simulink model "GalacticSoupPhysical"  (R2025b)
settings: Solver=VariableStepAuto  StartTime=0.0  StopTime=10.0  RelTol=1e-3
settings Model: DataDictionary=GalacticSoupPhysicalInterfaces.sldd  Creator=sarah  LastModifiedBy=sarah

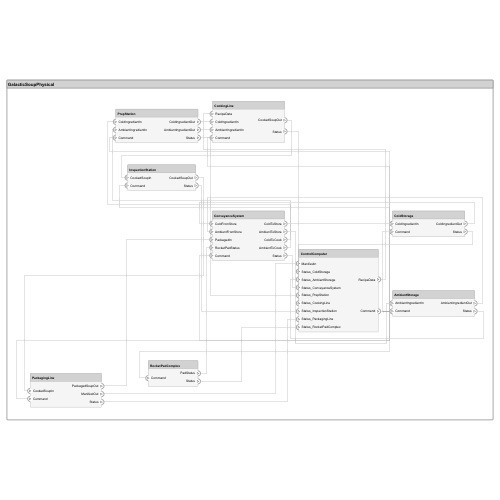
[thumbnail: Simulink's stored preview of the top-level diagram]
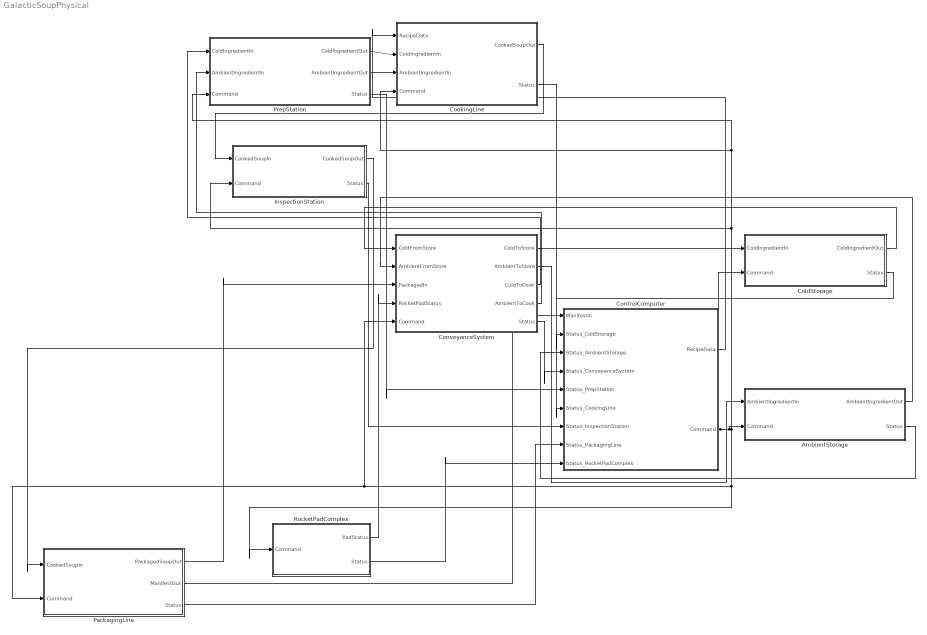
== system GalacticSoupPhysical ==
  AmbientStorage : Subsystem
      settings: PortSchema="{\"entries\":[{\"content\":{\"headerSize\":26,\"margin\":15,\"minimumSpacing\":25,\"sides\":[{\"content\":{\"connectorIds\":[\"In1\",\"In2\"]},\"type\":\"ConnectorPlacement.EquallySpacedRectSide\",\"uuid\":\"47548036-a6c3-440f-b573-2a4e753e82ae\"},{\"content\":{\"connectorIds\":[\"Out1\",\"Out2\"],\"side\":\"RIGHT\"},\"type\":\"ConnectorPlacement.EquallySpacedRectSide\",\"uuid\":\"ab096620-2054-4429-8520-52cfe6541bb8\"},{\"content\":{\"side\":\"TOP\"},\"type\":\"ConnectorPlacement.EquallySpacedRectSide\",\"uuid\":\"6e18e29c-ba68-48ca-8847-f496b38e15b5\"}]},\"type\":\"ConnectorPlacement.EquallySpacedConnector\",\"uuid\":\"7233fc04-a641-40d9-8870-909b934a9733\"}],\"packageUris\":[\"http://schema.mathworks.com/mf0/Connector/R2020b\"],\"version\":\"1.0\"}"
  ColdStorage : Subsystem
      settings: PortSchema="{\"entries\":[{\"content\":{\"headerSize\":26,\"margin\":15,\"minimumSpacing\":25,\"sides\":[{\"content\":{\"connectorIds\":[\"In1\",\"In2\"]},\"type\":\"ConnectorPlacement.EquallySpacedRectSide\",\"uuid\":\"47548036-a6c3-440f-b573-2a4e753e82ae\"},{\"content\":{\"connectorIds\":[\"Out1\",\"Out2\"],\"side\":\"RIGHT\"},\"type\":\"ConnectorPlacement.EquallySpacedRectSide\",\"uuid\":\"ab096620-2054-4429-8520-52cfe6541bb8\"},{\"content\":{\"side\":\"TOP\"},\"type\":\"ConnectorPlacement.EquallySpacedRectSide\",\"uuid\":\"6e18e29c-ba68-48ca-8847-f496b38e15b5\"}]},\"type\":\"ConnectorPlacement.EquallySpacedConnector\",\"uuid\":\"7233fc04-a641-40d9-8870-909b934a9733\"}],\"packageUris\":[\"http://schema.mathworks.com/mf0/Connector/R2020b\"],\"version\":\"1.0\"}"
  ControlComputer : Subsystem
      settings: PortSchema="{\"entries\":[{\"content\":{\"headerSize\":26,\"margin\":15,\"minimumSpacing\":25,\"sides\":[{\"content\":{\"connectorIds\":[\"In1\",\"In2\",\"In3\",\"In4\",\"In5\",\"In6\",\"In7\",\"In8\",\"In9\"]},\"type\":\"ConnectorPlacement.EquallySpacedRectSide\",\"uuid\":\"47548036-a6c3-440f-b573-2a4e753e82ae\"},{\"content\":{\"connectorIds\":[\"Out1\",\"Out2\"],\"side\":\"RIGHT\"},\"type\":\"ConnectorPlacement.EquallySpacedRectSide\",\"uuid\":\"ab096620-2054-4429-8520-52cfe6541bb8\"},{\"content\":{\"side\":\"TOP\"},\"type\":\"ConnectorPlacement.EquallySpacedRectSide\",\"uuid\":\"6e18e29c-ba68-48ca-8847-f496b38e15b5\"}]},\"type\":\"ConnectorPlacement.EquallySpacedConnector\",\"uuid\":\"7233fc04-a641-40d9-8870-909b934a9733\"}],\"packageUris\":[\"http://schema.mathworks.com/mf0/Connector/R2020b\"],\"version\":\"1.0\"}"
  ConveyanceSystem : Subsystem
      settings: PortSchema="{\"entries\":[{\"content\":{\"headerSize\":26,\"margin\":15,\"minimumSpacing\":25,\"sides\":[{\"content\":{\"connectorIds\":[\"In1\",\"In2\",\"In3\",\"In4\",\"In5\"]},\"type\":\"ConnectorPlacement.EquallySpacedRectSide\",\"uuid\":\"47548036-a6c3-440f-b573-2a4e753e82ae\"},{\"content\":{\"connectorIds\":[\"Out1\",\"Out2\",\"Out3\",\"Out4\",\"Out5\"],\"side\":\"RIGHT\"},\"type\":\"ConnectorPlacement.EquallySpacedRectSide\",\"uuid\":\"ab096620-2054-4429-8520-52cfe6541bb8\"},{\"content\":{\"side\":\"TOP\"},\"type\":\"ConnectorPlacement.EquallySpacedRectSide\",\"uuid\":\"6e18e29c-ba68-48ca-8847-f496b38e15b5\"}]},\"type\":\"ConnectorPlacement.EquallySpacedConnector\",\"uuid\":\"7233fc04-a641-40d9-8870-909b934a9733\"}],\"packageUris\":[\"http://schema.mathworks.com/mf0/Connector/R2020b\"],\"version\":\"1.0\"}"
  CookingLine : Subsystem
      settings: PortSchema="{\"entries\":[{\"content\":{\"headerSize\":26,\"margin\":15,\"minimumSpacing\":25,\"sides\":[{\"content\":{\"connectorIds\":[\"In1\",\"In2\",\"In3\",\"In4\"]},\"type\":\"ConnectorPlacement.EquallySpacedRectSide\",\"uuid\":\"47548036-a6c3-440f-b573-2a4e753e82ae\"},{\"content\":{\"connectorIds\":[\"Out1\",\"Out2\"],\"side\":\"RIGHT\"},\"type\":\"ConnectorPlacement.EquallySpacedRectSide\",\"uuid\":\"ab096620-2054-4429-8520-52cfe6541bb8\"},{\"content\":{\"side\":\"TOP\"},\"type\":\"ConnectorPlacement.EquallySpacedRectSide\",\"uuid\":\"6e18e29c-ba68-48ca-8847-f496b38e15b5\"}]},\"type\":\"ConnectorPlacement.EquallySpacedConnector\",\"uuid\":\"7233fc04-a641-40d9-8870-909b934a9733\"}],\"packageUris\":[\"http://schema.mathworks.com/mf0/Connector/R2020b\"],\"version\":\"1.0\"}"
  InspectionStation : Subsystem
      settings: PortSchema="{\"entries\":[{\"content\":{\"headerSize\":26,\"margin\":15,\"minimumSpacing\":25,\"sides\":[{\"content\":{\"connectorIds\":[\"In1\",\"In2\"]},\"type\":\"ConnectorPlacement.EquallySpacedRectSide\",\"uuid\":\"47548036-a6c3-440f-b573-2a4e753e82ae\"},{\"content\":{\"connectorIds\":[\"Out1\",\"Out2\"],\"side\":\"RIGHT\"},\"type\":\"ConnectorPlacement.EquallySpacedRectSide\",\"uuid\":\"ab096620-2054-4429-8520-52cfe6541bb8\"},{\"content\":{\"side\":\"TOP\"},\"type\":\"ConnectorPlacement.EquallySpacedRectSide\",\"uuid\":\"6e18e29c-ba68-48ca-8847-f496b38e15b5\"}]},\"type\":\"ConnectorPlacement.EquallySpacedConnector\",\"uuid\":\"7233fc04-a641-40d9-8870-909b934a9733\"}],\"packageUris\":[\"http://schema.mathworks.com/mf0/Connector/R2020b\"],\"version\":\"1.0\"}"
  PackagingLine : Subsystem
      settings: PortSchema="{\"entries\":[{\"content\":{\"headerSize\":26,\"margin\":15,\"minimumSpacing\":25,\"sides\":[{\"content\":{\"connectorIds\":[\"In1\",\"In2\"]},\"type\":\"ConnectorPlacement.EquallySpacedRectSide\",\"uuid\":\"47548036-a6c3-440f-b573-2a4e753e82ae\"},{\"content\":{\"connectorIds\":[\"Out1\",\"Out2\",\"Out3\"],\"side\":\"RIGHT\"},\"type\":\"ConnectorPlacement.EquallySpacedRectSide\",\"uuid\":\"ab096620-2054-4429-8520-52cfe6541bb8\"},{\"content\":{\"side\":\"TOP\"},\"type\":\"ConnectorPlacement.EquallySpacedRectSide\",\"uuid\":\"6e18e29c-ba68-48ca-8847-f496b38e15b5\"}]},\"type\":\"ConnectorPlacement.EquallySpacedConnector\",\"uuid\":\"7233fc04-a641-40d9-8870-909b934a9733\"}],\"packageUris\":[\"http://schema.mathworks.com/mf0/Connector/R2020b\"],\"version\":\"1.0\"}"
  PrepStation : Subsystem
      settings: PortSchema="{\"entries\":[{\"content\":{\"headerSize\":26,\"margin\":15,\"minimumSpacing\":25,\"sides\":[{\"content\":{\"connectorIds\":[\"In1\",\"In2\",\"In3\"]},\"type\":\"ConnectorPlacement.EquallySpacedRectSide\",\"uuid\":\"47548036-a6c3-440f-b573-2a4e753e82ae\"},{\"content\":{\"connectorIds\":[\"Out1\",\"Out2\",\"Out3\"],\"side\":\"RIGHT\"},\"type\":\"ConnectorPlacement.EquallySpacedRectSide\",\"uuid\":\"ab096620-2054-4429-8520-52cfe6541bb8\"},{\"content\":{\"side\":\"TOP\"},\"type\":\"ConnectorPlacement.EquallySpacedRectSide\",\"uuid\":\"6e18e29c-ba68-48ca-8847-f496b38e15b5\"}]},\"type\":\"ConnectorPlacement.EquallySpacedConnector\",\"uuid\":\"7233fc04-a641-40d9-8870-909b934a9733\"}],\"packageUris\":[\"http://schema.mathworks.com/mf0/Connector/R2020b\"],\"version\":\"1.0\"}"
  RocketPadComplex : Subsystem
      settings: PortSchema="{\"entries\":[{\"content\":{\"headerSize\":26,\"margin\":15,\"minimumSpacing\":25,\"sides\":[{\"content\":{\"connectorIds\":[\"In1\"]},\"type\":\"ConnectorPlacement.EquallySpacedRectSide\",\"uuid\":\"47548036-a6c3-440f-b573-2a4e753e82ae\"},{\"content\":{\"connectorIds\":[\"Out1\",\"Out2\"],\"side\":\"RIGHT\"},\"type\":\"ConnectorPlacement.EquallySpacedRectSide\",\"uuid\":\"ab096620-2054-4429-8520-52cfe6541bb8\"},{\"content\":{\"side\":\"TOP\"},\"type\":\"ConnectorPlacement.EquallySpacedRectSide\",\"uuid\":\"6e18e29c-ba68-48ca-8847-f496b38e15b5\"}]},\"type\":\"ConnectorPlacement.EquallySpacedConnector\",\"uuid\":\"7233fc04-a641-40d9-8870-909b934a9733\"}],\"packageUris\":[\"http://schema.mathworks.com/mf0/Connector/R2020b\"],\"version\":\"1.0\"}"
  wires:
  RocketPadComplex/2(Status) -> ControlComputer/9(Status_RocketPadComplex)
  PrepStation/2(AmbientIngredientOut) -> CookingLine/3(AmbientIngredientIn)
  InspectionStation/1(CookedSoupOut) -> PackagingLine/1(CookedSoupIn)
  InspectionStation/2(Status) -> ControlComputer/7(Status_InspectionStation)
  PackagingLine/3(Status) -> ControlComputer/8(Status_PackagingLine)
  PackagingLine/1(PackagedSoupOut) -> ConveyanceSystem/3(PackagedIn)
  PackagingLine/2(ManifestOut) -> ControlComputer/1(ManifestIn)
  PrepStation/1(ColdIngredientOut) -> CookingLine/2(ColdIngredientIn)
  PrepStation/3(Status) -> ControlComputer/5(Status_PrepStation)
  RocketPadComplex/1(PadStatus) -> ConveyanceSystem/4(RocketPadStatus)
  CookingLine/1(CookedSoupOut) -> InspectionStation/1(CookedSoupIn)
  CookingLine/2(Status) -> ControlComputer/6(Status_CookingLine)
  ConveyanceSystem/1(ColdToStore) -> ColdStorage/1(ColdIngredientIn)
  ConveyanceSystem/2(AmbientToStore) -> AmbientStorage/1(AmbientIngredientIn)
  ConveyanceSystem/4(AmbientToCook) -> PrepStation/2(AmbientIngredientIn)
  ConveyanceSystem/3(ColdToCook) -> PrepStation/1(ColdIngredientIn)
  ConveyanceSystem/5(Status) -> ControlComputer/4(Status_ConveyanceSystem)
  ControlComputer/2(Command) -> PackagingLine/2(Command), ConveyanceSystem/5(Command), RocketPadComplex/1(Command), CookingLine/4(Command), PrepStation/3(Command), InspectionStation/2(Command), AmbientStorage/2(Command), ColdStorage/2(Command)
  ControlComputer/1(RecipeData) -> CookingLine/1(RecipeData)
  ColdStorage/1(ColdIngredientOut) -> ConveyanceSystem/1(ColdFromStore)
  ColdStorage/2(Status) -> ControlComputer/2(Status_ColdStorage)
  AmbientStorage/1(AmbientIngredientOut) -> ConveyanceSystem/2(AmbientFromStore)
  AmbientStorage/2(Status) -> ControlComputer/3(Status_AmbientStorage)

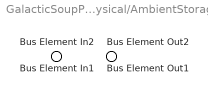
== system GalacticSoupPhysical/AmbientStorage ==
  Bus Element In1 : Inport  PortName=AmbientIngredientIn
  Bus Element In2 : Inport  Port=2  PortName=Command
  Bus Element Out1 : Outport  PortName=AmbientIngredientOut
  Bus Element Out2 : Outport  Port=2  PortName=Status

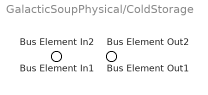
== system GalacticSoupPhysical/ColdStorage ==
  Bus Element In1 : Inport  PortName=ColdIngredientIn
  Bus Element In2 : Inport  Port=2  PortName=Command
  Bus Element Out1 : Outport  PortName=ColdIngredientOut
  Bus Element Out2 : Outport  Port=2  PortName=Status

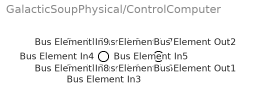
== system GalacticSoupPhysical/ControlComputer ==
  Bus Element In1 : Inport  PortName=ManifestIn
  Bus Element In2 : Inport  Port=2  PortName=Status_ColdStorage
  Bus Element In3 : Inport  Port=3  PortName=Status_AmbientStorage
  Bus Element In4 : Inport  Port=4  PortName=Status_ConveyanceSystem
  Bus Element In5 : Inport  Port=5  PortName=Status_PrepStation
  Bus Element In6 : Inport  Port=6  PortName=Status_CookingLine
  Bus Element In7 : Inport  Port=7  PortName=Status_InspectionStation
  Bus Element In8 : Inport  Port=8  PortName=Status_PackagingLine
  Bus Element In9 : Inport  Port=9  PortName=Status_RocketPadComplex
  Bus Element Out1 : Outport  PortName=RecipeData
  Bus Element Out2 : Outport  Port=2  PortName=Command

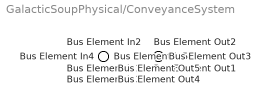
== system GalacticSoupPhysical/ConveyanceSystem ==
  Bus Element In1 : Inport  PortName=ColdFromStore
  Bus Element In2 : Inport  Port=2  PortName=AmbientFromStore
  Bus Element In3 : Inport  Port=3  PortName=PackagedIn
  Bus Element In4 : Inport  Port=4  PortName=RocketPadStatus
  Bus Element In5 : Inport  Port=5  PortName=Command
  Bus Element Out1 : Outport  PortName=ColdToStore
  Bus Element Out2 : Outport  Port=2  PortName=AmbientToStore
  Bus Element Out3 : Outport  Port=3  PortName=ColdToCook
  Bus Element Out4 : Outport  Port=4  PortName=AmbientToCook
  Bus Element Out5 : Outport  Port=5  PortName=Status

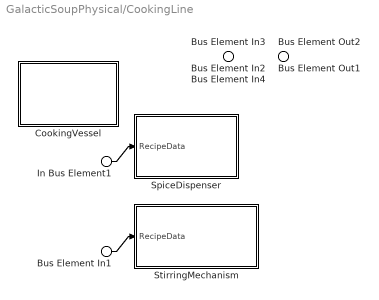
== system GalacticSoupPhysical/CookingLine ==
  Bus Element In1 : Inport  PortName=RecipeData
  In Bus Element1 : Inport  PortName=RecipeData
  Bus Element In2 : Inport  Port=2  PortName=ColdIngredientIn
  Bus Element In3 : Inport  Port=3  PortName=AmbientIngredientIn
  Bus Element In4 : Inport  Port=4  PortName=Command
  CookingVessel : Subsystem
      settings: PortSchema="{\"entries\":[{\"content\":{\"headerSize\":26,\"margin\":15,\"minimumSpacing\":25,\"sides\":[{\"content\":{},\"type\":\"ConnectorPlacement.EquallySpacedRectSide\",\"uuid\":\"47548036-a6c3-440f-b573-2a4e753e82ae\"},{\"content\":{\"side\":\"RIGHT\"},\"type\":\"ConnectorPlacement.EquallySpacedRectSide\",\"uuid\":\"ab096620-2054-4429-8520-52cfe6541bb8\"},{\"content\":{\"side\":\"TOP\"},\"type\":\"ConnectorPlacement.EquallySpacedRectSide\",\"uuid\":\"6e18e29c-ba68-48ca-8847-f496b38e15b5\"}]},\"type\":\"ConnectorPlacement.EquallySpacedConnector\",\"uuid\":\"7233fc04-a641-40d9-8870-909b934a9733\"}],\"packageUris\":[\"http://schema.mathworks.com/mf0/Connector/R2020b\"],\"version\":\"1.0\"}"
  SpiceDispenser : Subsystem
      settings: PortSchema="{\"entries\":[{\"content\":{\"headerSize\":26,\"margin\":15,\"minimumSpacing\":25,\"sides\":[{\"content\":{\"connectorIds\":[\"In1\"]},\"type\":\"ConnectorPlacement.EquallySpacedRectSide\",\"uuid\":\"47548036-a6c3-440f-b573-2a4e753e82ae\"},{\"content\":{\"side\":\"RIGHT\"},\"type\":\"ConnectorPlacement.EquallySpacedRectSide\",\"uuid\":\"ab096620-2054-4429-8520-52cfe6541bb8\"},{\"content\":{\"side\":\"TOP\"},\"type\":\"ConnectorPlacement.EquallySpacedRectSide\",\"uuid\":\"6e18e29c-ba68-48ca-8847-f496b38e15b5\"}]},\"type\":\"ConnectorPlacement.EquallySpacedConnector\",\"uuid\":\"7233fc04-a641-40d9-8870-909b934a9733\"}],\"packageUris\":[\"http://schema.mathworks.com/mf0/Connector/R2020b\"],\"version\":\"1.0\"}"
  StirringMechanism : Subsystem
      settings: PortSchema="{\"entries\":[{\"content\":{\"headerSize\":26,\"margin\":15,\"minimumSpacing\":25,\"sides\":[{\"content\":{\"connectorIds\":[\"In1\"]},\"type\":\"ConnectorPlacement.EquallySpacedRectSide\",\"uuid\":\"47548036-a6c3-440f-b573-2a4e753e82ae\"},{\"content\":{\"side\":\"RIGHT\"},\"type\":\"ConnectorPlacement.EquallySpacedRectSide\",\"uuid\":\"ab096620-2054-4429-8520-52cfe6541bb8\"},{\"content\":{\"side\":\"TOP\"},\"type\":\"ConnectorPlacement.EquallySpacedRectSide\",\"uuid\":\"6e18e29c-ba68-48ca-8847-f496b38e15b5\"}]},\"type\":\"ConnectorPlacement.EquallySpacedConnector\",\"uuid\":\"7233fc04-a641-40d9-8870-909b934a9733\"}],\"packageUris\":[\"http://schema.mathworks.com/mf0/Connector/R2020b\"],\"version\":\"1.0\"}"
  Bus Element Out1 : Outport  PortName=CookedSoupOut
  Bus Element Out2 : Outport  Port=2  PortName=Status
  wires:
  In Bus Element1/1 -> SpiceDispenser/1(RecipeData)
  Bus Element In1/1 -> StirringMechanism/1(RecipeData)

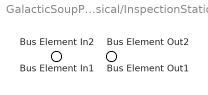
== system GalacticSoupPhysical/InspectionStation ==
  Bus Element In1 : Inport  PortName=CookedSoupIn
  Bus Element In2 : Inport  Port=2  PortName=Command
  Bus Element Out1 : Outport  PortName=CookedSoupOut
  Bus Element Out2 : Outport  Port=2  PortName=Status

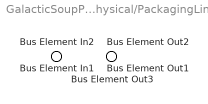
== system GalacticSoupPhysical/PackagingLine ==
  Bus Element In1 : Inport  PortName=CookedSoupIn
  Bus Element In2 : Inport  Port=2  PortName=Command
  Bus Element Out1 : Outport  PortName=PackagedSoupOut
  Bus Element Out2 : Outport  Port=2  PortName=ManifestOut
  Bus Element Out3 : Outport  Port=3  PortName=Status

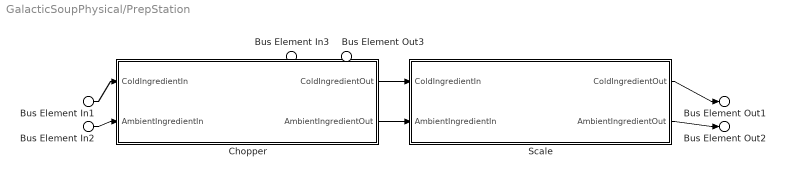
== system GalacticSoupPhysical/PrepStation ==
  Bus Element In1 : Inport  PortName=ColdIngredientIn
  Bus Element In2 : Inport  Port=2  PortName=AmbientIngredientIn
  Bus Element In3 : Inport  Port=3  PortName=Command
  Chopper : Subsystem
      settings: PortSchema="{\"entries\":[{\"content\":{\"headerSize\":26,\"margin\":15,\"minimumSpacing\":25,\"sides\":[{\"content\":{\"connectorIds\":[\"In1\",\"In2\"]},\"type\":\"ConnectorPlacement.EquallySpacedRectSide\",\"uuid\":\"47548036-a6c3-440f-b573-2a4e753e82ae\"},{\"content\":{\"connectorIds\":[\"Out1\",\"Out2\"],\"side\":\"RIGHT\"},\"type\":\"ConnectorPlacement.EquallySpacedRectSide\",\"uuid\":\"ab096620-2054-4429-8520-52cfe6541bb8\"},{\"content\":{\"side\":\"TOP\"},\"type\":\"ConnectorPlacement.EquallySpacedRectSide\",\"uuid\":\"6e18e29c-ba68-48ca-8847-f496b38e15b5\"}]},\"type\":\"ConnectorPlacement.EquallySpacedConnector\",\"uuid\":\"7233fc04-a641-40d9-8870-909b934a9733\"}],\"packageUris\":[\"http://schema.mathworks.com/mf0/Connector/R2020b\"],\"version\":\"1.0\"}"
  Scale : Subsystem
      settings: PortSchema="{\"entries\":[{\"content\":{\"headerSize\":26,\"margin\":15,\"minimumSpacing\":25,\"sides\":[{\"content\":{\"connectorIds\":[\"In1\",\"In2\"]},\"type\":\"ConnectorPlacement.EquallySpacedRectSide\",\"uuid\":\"47548036-a6c3-440f-b573-2a4e753e82ae\"},{\"content\":{\"connectorIds\":[\"Out1\",\"Out2\"],\"side\":\"RIGHT\"},\"type\":\"ConnectorPlacement.EquallySpacedRectSide\",\"uuid\":\"ab096620-2054-4429-8520-52cfe6541bb8\"},{\"content\":{\"side\":\"TOP\"},\"type\":\"ConnectorPlacement.EquallySpacedRectSide\",\"uuid\":\"6e18e29c-ba68-48ca-8847-f496b38e15b5\"}]},\"type\":\"ConnectorPlacement.EquallySpacedConnector\",\"uuid\":\"7233fc04-a641-40d9-8870-909b934a9733\"}],\"packageUris\":[\"http://schema.mathworks.com/mf0/Connector/R2020b\"],\"version\":\"1.0\"}"
  Bus Element Out1 : Outport  PortName=ColdIngredientOut
  Bus Element Out2 : Outport  Port=2  PortName=AmbientIngredientOut
  Bus Element Out3 : Outport  Port=3  PortName=Status
  wires:
  Bus Element In1/1 -> Chopper/1(ColdIngredientIn)
  Bus Element In2/1 -> Chopper/2(AmbientIngredientIn)
  Scale/1(ColdIngredientOut) -> Bus Element Out1/1
  Chopper/1(ColdIngredientOut) -> Scale/1(ColdIngredientIn)
  Chopper/2(AmbientIngredientOut) -> Scale/2(AmbientIngredientIn)
  Scale/2(AmbientIngredientOut) -> Bus Element Out2/1

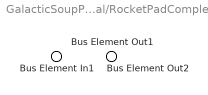
== system GalacticSoupPhysical/RocketPadComplex ==
  Bus Element In1 : Inport  PortName=Command
  Bus Element Out1 : Outport  PortName=PadStatus
  Bus Element Out2 : Outport  Port=2  PortName=Status

== system GalacticSoupPhysical/CookingLine/CookingVessel ==

== system GalacticSoupPhysical/CookingLine/SpiceDispenser ==
  Bus Element In1 : Inport  PortName=RecipeData

== system GalacticSoupPhysical/CookingLine/StirringMechanism ==
  Bus Element In1 : Inport  PortName=RecipeData

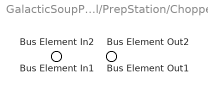
== system GalacticSoupPhysical/PrepStation/Chopper ==
  Bus Element In1 : Inport  PortName=ColdIngredientIn
  Bus Element In2 : Inport  Port=2  PortName=AmbientIngredientIn
  Bus Element Out1 : Outport  PortName=ColdIngredientOut
  Bus Element Out2 : Outport  Port=2  PortName=AmbientIngredientOut

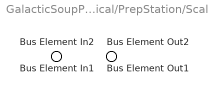
== system GalacticSoupPhysical/PrepStation/Scale ==
  Bus Element In1 : Inport  PortName=ColdIngredientIn
  Bus Element In2 : Inport  Port=2  PortName=AmbientIngredientIn
  Bus Element Out1 : Outport  PortName=ColdIngredientOut
  Bus Element Out2 : Outport  Port=2  PortName=AmbientIngredientOut
